simulink model "q4"  (R2024b)
settings: Solver=VariableStepAuto  StartTime=0.0  StopTime=5  RelTol=1e-3
settings Model: Creator=32602  LastModifiedBy=32602

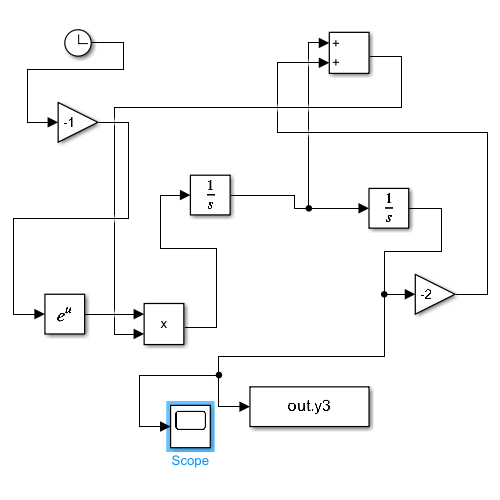
[thumbnail: Simulink's stored preview of the top-level diagram]
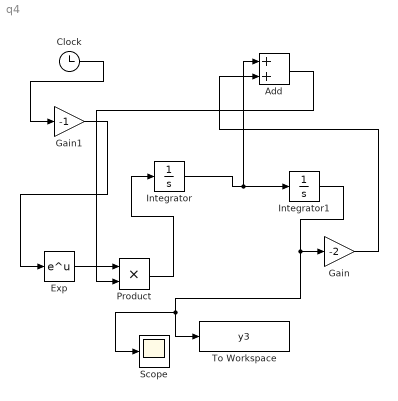
== system q4 ==
  Add : Sum
  Clock : Clock
  Exp : Math
  Gain : Gain  Gain=-2
  Gain1 : Gain  Gain=-1
  Integrator : Integrator  InitialCondition=1
  Integrator1 : Integrator
  Product : Product
  Scope : Scope
  To Workspace : ToWorkspace  VariableName=y3  SaveFormat=Timeseries  SampleTime=-1
  wires:
  Integrator/1 -> Add/1, Integrator1/1
  Integrator1/1 -> To Workspace/1, Scope/1, Gain/1
  Gain/1 -> Add/2
  Clock/1 -> Gain1/1
  Gain1/1 -> Exp/1
  Exp/1 -> Product/1
  Add/1 -> Product/2
  Product/1 -> Integrator/1
